simulink model "Motor_Model_full"  (R2015b)
settings: Solver=VariableStepAuto  StartTime=0.0  StopTime=0.5  RelTol=1e-3
values from neighbouring files (symbols this model uses):
  pre_speed = 50    [motor_PI_Controller.m]
libraries: PIcontroller x13
settings Model: Creator=qlong1505  LastModifiedBy=s3358327

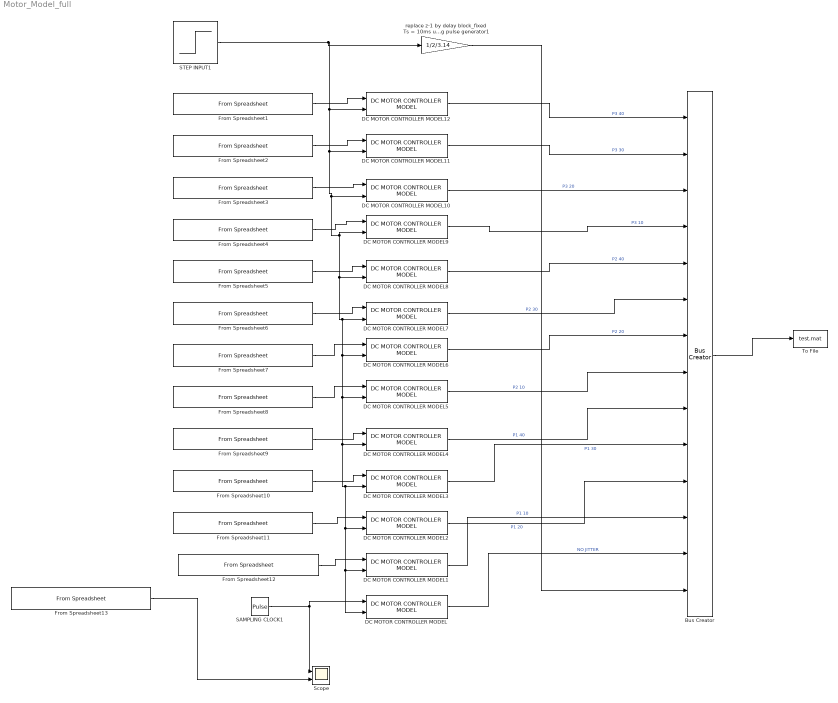
== system Motor_Model_full ==
  Bus Creator : BusCreator  Inputs=14
  DC MOTOR CONTROLLER MODEL{,1..12} (13 alike) : PIcontroller/DC MOTOR CONTROLLER MODEL
  From Spreadsheet1 : FromSpreadsheet  FileName=pattern.xlsx  SheetName=P3_40  OutDataTypeStr=double  SampleTime=0.0001  ExtrapolationBeforeFirstDataPoint=Ground value  InterpolationWithinTimeRange=Zero order hold
  From Spreadsheet10 : FromSpreadsheet  FileName=pattern.xlsx  SheetName=P1_30  OutDataTypeStr=double  SampleTime=0.0001  ExtrapolationBeforeFirstDataPoint=Ground value  InterpolationWithinTimeRange=Zero order hold
  From Spreadsheet11 : FromSpreadsheet  FileName=pattern.xlsx  SheetName=P1_20  OutDataTypeStr=double  SampleTime=0.0001  ExtrapolationBeforeFirstDataPoint=Ground value  InterpolationWithinTimeRange=Zero order hold
  From Spreadsheet12 : FromSpreadsheet  FileName=pattern.xlsx  SheetName=P1_10  OutDataTypeStr=double  SampleTime=0.0001  ExtrapolationBeforeFirstDataPoint=Ground value  InterpolationWithinTimeRange=Zero order hold
  From Spreadsheet13 : FromSpreadsheet  FileName=pattern.xlsx  SheetName=No_jitter  OutDataTypeStr=double  SampleTime=0.0001  ExtrapolationBeforeFirstDataPoint=Ground value  InterpolationWithinTimeRange=Zero order hold
  From Spreadsheet2 : FromSpreadsheet  FileName=pattern.xlsx  SheetName=P3_30  OutDataTypeStr=double  SampleTime=0.0001  ExtrapolationBeforeFirstDataPoint=Ground value  InterpolationWithinTimeRange=Zero order hold
  From Spreadsheet3 : FromSpreadsheet  FileName=pattern.xlsx  SheetName=P3_20  OutDataTypeStr=double  SampleTime=0.0001  ExtrapolationBeforeFirstDataPoint=Ground value  InterpolationWithinTimeRange=Zero order hold
  From Spreadsheet4 : FromSpreadsheet  FileName=pattern.xlsx  SheetName=P3_10  OutDataTypeStr=double  SampleTime=0.0001  ExtrapolationBeforeFirstDataPoint=Ground value  InterpolationWithinTimeRange=Zero order hold
  From Spreadsheet5 : FromSpreadsheet  FileName=pattern.xlsx  SheetName=P2_40  OutDataTypeStr=double  SampleTime=0.0001  ExtrapolationBeforeFirstDataPoint=Ground value  InterpolationWithinTimeRange=Zero order hold
  From Spreadsheet6 : FromSpreadsheet  FileName=pattern.xlsx  SheetName=P2_30  OutDataTypeStr=double  SampleTime=0.0001  ExtrapolationBeforeFirstDataPoint=Ground value  InterpolationWithinTimeRange=Zero order hold
  From Spreadsheet7 : FromSpreadsheet  FileName=pattern.xlsx  SheetName=P2_20  OutDataTypeStr=double  SampleTime=0.0001  ExtrapolationBeforeFirstDataPoint=Ground value  InterpolationWithinTimeRange=Zero order hold
  From Spreadsheet8 : FromSpreadsheet  FileName=pattern.xlsx  SheetName=P2_10  OutDataTypeStr=double  SampleTime=0.0001  ExtrapolationBeforeFirstDataPoint=Ground value  InterpolationWithinTimeRange=Zero order hold
  From Spreadsheet9 : FromSpreadsheet  FileName=pattern.xlsx  SheetName=P1_40  OutDataTypeStr=double  SampleTime=0.0001  ExtrapolationBeforeFirstDataPoint=Ground value  InterpolationWithinTimeRange=Zero order hold
  SAMPLING CLOCK1 : DiscretePulseGenerator  PulseType=Time based  Period=0.01  PulseWidth=50
  STEP INPUT1 : Step  Time=0.2  Before=11*2*3.14  After=pre_speed*2*3.14  SampleTime=0
  Scope : Scope  NumInputPorts=2
  To File : ToFile  Filename=test.mat
  replace z-1 by delay block_fixed Ts = 10ms using pulse generator1 : Gain  Gain=1/2/3.14
  wires:
  DC MOTOR CONTROLLER MODEL1/1 -> Bus Creator/12  "P1 10"
  Bus Creator/1 -> To File/1
  DC MOTOR CONTROLLER MODEL2/1 -> Bus Creator/11  "P1 20"
  DC MOTOR CONTROLLER MODEL6/1 -> Bus Creator/7  "P2 20"
  DC MOTOR CONTROLLER MODEL5/1 -> Bus Creator/8  "P2 10"
  DC MOTOR CONTROLLER MODEL4/1 -> Bus Creator/9  "P1 40"
  DC MOTOR CONTROLLER MODEL3/1 -> Bus Creator/10  "P1 30"
  DC MOTOR CONTROLLER MODEL9/1 -> Bus Creator/4  "P3 10"
  DC MOTOR CONTROLLER MODEL8/1 -> Bus Creator/5  "P2 40"
  DC MOTOR CONTROLLER MODEL7/1 -> Bus Creator/6  "P2 30"
  DC MOTOR CONTROLLER MODEL10/1 -> Bus Creator/3  "P3 20"
  DC MOTOR CONTROLLER MODEL11/1 -> Bus Creator/2  "P3 30"
  DC MOTOR CONTROLLER MODEL12/1 -> Bus Creator/1  "P3 40"
  DC MOTOR CONTROLLER MODEL/1 -> Bus Creator/13  "NO JITTER"
  From Spreadsheet1/1 -> DC MOTOR CONTROLLER MODEL12/1
  From Spreadsheet2/1 -> DC MOTOR CONTROLLER MODEL11/1
  From Spreadsheet3/1 -> DC MOTOR CONTROLLER MODEL10/1
  From Spreadsheet4/1 -> DC MOTOR CONTROLLER MODEL9/1
  From Spreadsheet5/1 -> DC MOTOR CONTROLLER MODEL8/1
  From Spreadsheet6/1 -> DC MOTOR CONTROLLER MODEL7/1
  From Spreadsheet7/1 -> DC MOTOR CONTROLLER MODEL6/1
  From Spreadsheet8/1 -> DC MOTOR CONTROLLER MODEL5/1
  From Spreadsheet9/1 -> DC MOTOR CONTROLLER MODEL4/1
  From Spreadsheet10/1 -> DC MOTOR CONTROLLER MODEL3/1
  From Spreadsheet11/1 -> DC MOTOR CONTROLLER MODEL2/1
  From Spreadsheet12/1 -> DC MOTOR CONTROLLER MODEL1/1
  STEP INPUT1/1 -> replace z-1 by delay block_fixed Ts = 10ms using pulse generator1/1, DC MOTOR CONTROLLER MODEL12/2, DC MOTOR CONTROLLER MODEL11/2, DC MOTOR CONTROLLER MODEL10/2, DC MOTOR CONTROLLER MODEL9/2, DC MOTOR CONTROLLER MODEL8/2, DC MOTOR CONTROLLER MODEL7/2, DC MOTOR CONTROLLER MODEL6/2, DC MOTOR CONTROLLER MODEL4/2, DC MOTOR CONTROLLER MODEL3/2, DC MOTOR CONTROLLER MODEL2/2, DC MOTOR CONTROLLER MODEL1/2, DC MOTOR CONTROLLER MODEL/2, DC MOTOR CONTROLLER MODEL5/2
  replace z-1 by delay block_fixed Ts = 10ms using pulse generator1/1 -> Bus Creator/14
  From Spreadsheet13/1 -> Scope/2
  SAMPLING CLOCK1/1 -> Scope/1, DC MOTOR CONTROLLER MODEL/1
